simulink subsystem "FuelCellCore"  (R2023b)
settings: Solver=VariableStepAuto  StartTime=0.0  StopTime=10.0  RelTol=1e-3
undefined symbols (not defined in the file): anode_tube_D, cathode_tube_D, comp_rpm_TLU, coolant_num_layers, coolant_num_passes, coolant_tube_D, coolant_w_channels, env_p, env_T, N2_T, radiator_air_area_fins, radiator_air_area_primary, radiator_eta_fin, radiator_N_tubes, radiator_rho, radiator_t_wall, radiator_tube_H, radiator_W, stack_area, stack_iL, stack_mea_rho, stack_num_cells, stack_num_channels, stack_t_gdl, stack_t_membrane, stack_w_channels
libraries: fl_lib x98, nesl_utility_internal x20, slpidlib x2
(part 1 of 3)
settings Model: ModifiedByFormat=The MathWorks, Inc.  Creator=The MathWorks, Inc.  LastModifiedBy=The MathWorks, Inc.
settings SolverCC: MaxZcPerStep=1
settings OptimizationCC: ReuseModelBlockBuffer=off
settings DebuggingCC: UnconnectedInputMsg=warning  UnconnectedOutputMsg=warning  UnconnectedLineMsg=warning  SubsystemReferenceDiagnosticForUnitTest=warning
settings ModelReferenceCC: EnableRefExpFcnMdlSchedulingChecks=on
settings RTWCC: DLArmComputeVersion=19.05

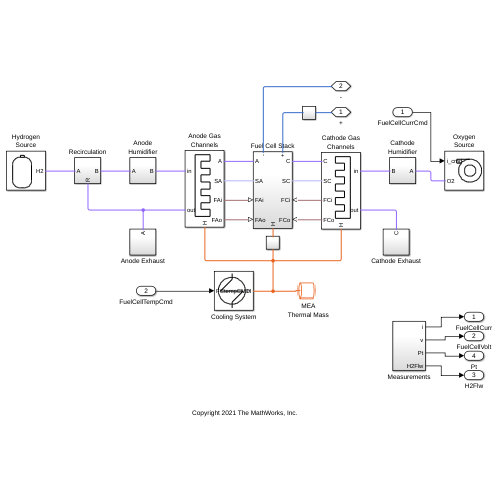
[thumbnail: Simulink's stored preview of the top-level diagram]
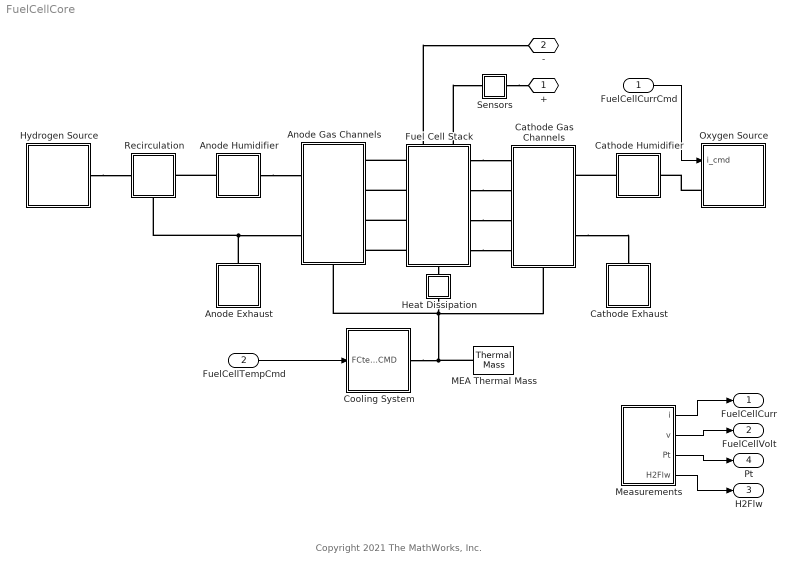
== system FuelCellCore ==
  note: Copyright 2021 The MathWorks, Inc.
  FuelCellCurrCmd : Inport
  FuelCellTempCmd : Inport  Port=2
  Anode Humidifier : Subsystem  Tag=PublishSubsystem
  Anode Exhaust : Subsystem  Tag=PublishSubsystem
      settings: PortSchema="{\"entries\":[{\"content\":{\"sides\":[{\"content\":{\"connectorIds\":[]},\"type\":\"ConnectorPlacement.EquallySpacedRectSide\",\"uuid\":\"6344d1cf-22ea-4a51-9588-07afca0fac15\"},{\"content\":{\"connectorIds\":[],\"side\":\"RIGHT\"},\"type\":\"ConnectorPlacement.EquallySpacedRectSide\",\"uuid\":\"a3908f81-9410-4056-87cd-9faba76d3fb8\"},{\"content\":{\"connectorIds\":[\"LConn1\"],\"side\":\"TOP\"},\"type\":\"ConnectorPlacement.EquallySpacedRectSide\",\"uuid\":\"a1c9e24d-adb9-4361-8e9b-feafccbbdb81\"}]},\"type\":\"ConnectorPlacement.EquallySpacedConnector\",\"uuid\":\"d5180d8f-18a0-491d-9fff-909db43c9aea\"}],\"packageUris\":[\"http://schema.mathworks.com/mf0/Connector/R2020b\"],\"version\":\"1.0\"}"
  Anode Gas Channels : Subsystem  Tag=PublishSubsystem
      settings: PortSchema="{\"entries\":[{\"content\":{\"sides\":[{\"content\":{\"connectorIds\":[\"LConn1\",\"LConn2\"]},\"type\":\"ConnectorPlacement.EquallySpacedRectSide\",\"uuid\":\"f0c92738-2de1-40ac-9e4a-670524600aa2\"},{\"content\":{\"connectorIds\":[\"RConn1\",\"RConn2\",\"RConn3\",\"RConn4\"],\"side\":\"RIGHT\"},\"type\":\"ConnectorPlacement.EquallySpacedRectSide\",\"uuid\":\"f0ed995d-2dce-4bd6-9faa-b1cb502a30b1\"},{\"content\":{\"connectorIds\":[],\"side\":\"TOP\"},\"type\":\"ConnectorPlacement.EquallySpacedRectSide\",\"uuid\":\"b5d2d698-46b6-42b5-a767-bb9f1790aa28\"},{\"content\":{\"connectorIds\":[\"RConn5\"],\"side\":\"BOTTOM\"},\"type\":\"ConnectorPlacement.EquallySpacedRectSide\",\"uuid\":\"3e8c99a3-0044-43a9-bacb-b652445e4ac6\"}]},\"type\":\"ConnectorPlacement.EquallySpacedConnector\",\"uuid\":\"912925fb-ca80-4fe6-8a1d-a2308cfd6f88\"}],\"packageUris\":[\"http://schema.mathworks.com/mf0/Connector/R2020b\"],\"version\":\"1.0\"}"
      mask Display:
      | plot(0, 0)
      | plot(100, 100)
      | 
      | x1 = 25;
      | x2 = 65;
      | y1 = 23;
      | y2 = 95;
      | xt = 15;
      | yt = 9;
      | 
      | x_pattern = [x2 x2    x1+xt x1+xt   x1+xt   x2     ];
      | y_pattern = [y2 y2-yt y2-yt y2-2*yt y2-2*yt y2-2*yt];
      | 
      | plot([x1 x1 x2 x_pattern x_pattern      x_pattern      x_pattern         x2    x1], ...
      |      [y1-yt y2 y2 y_pattern y_pattern-2*yt y_pattern-4*yt y_pattern-6*yt y1-yt y1-yt])
  Cathode Humidifier : Subsystem  Tag=PublishSubsystem
  Cathode Exhaust : Subsystem  Tag=PublishSubsystem
      settings: PortSchema="{\"entries\":[{\"content\":{\"sides\":[{\"content\":{\"connectorIds\":[]},\"type\":\"ConnectorPlacement.EquallySpacedRectSide\",\"uuid\":\"6344d1cf-22ea-4a51-9588-07afca0fac15\"},{\"content\":{\"connectorIds\":[],\"side\":\"RIGHT\"},\"type\":\"ConnectorPlacement.EquallySpacedRectSide\",\"uuid\":\"a3908f81-9410-4056-87cd-9faba76d3fb8\"},{\"content\":{\"connectorIds\":[\"LConn1\"],\"side\":\"TOP\"},\"type\":\"ConnectorPlacement.EquallySpacedRectSide\",\"uuid\":\"a1c9e24d-adb9-4361-8e9b-feafccbbdb81\"}]},\"type\":\"ConnectorPlacement.EquallySpacedConnector\",\"uuid\":\"d5180d8f-18a0-491d-9fff-909db43c9aea\"}],\"packageUris\":[\"http://schema.mathworks.com/mf0/Connector/R2020b\"],\"version\":\"1.0\"}"
  Cathode Gas Channels : Subsystem  Tag=PublishSubsystem
      settings: PortSchema="{\"entries\":[{\"content\":{\"sides\":[{\"content\":{\"connectorIds\":[\"LConn1\",\"LConn2\",\"LConn3\",\"LConn4\"]},\"type\":\"ConnectorPlacement.EquallySpacedRectSide\",\"uuid\":\"d09155df-6760-40de-80f3-d532399b6b43\"},{\"content\":{\"connectorIds\":[\"RConn1\",\"RConn2\"],\"side\":\"RIGHT\"},\"type\":\"ConnectorPlacement.EquallySpacedRectSide\",\"uuid\":\"8f76bd4e-30c2-4c8b-860a-78c10353bd22\"},{\"content\":{\"connectorIds\":[],\"side\":\"TOP\"},\"type\":\"ConnectorPlacement.EquallySpacedRectSide\",\"uuid\":\"7de91a32-4f26-479e-bbec-b6009a288b8f\"},{\"content\":{\"connectorIds\":[\"RConn3\"],\"side\":\"BOTTOM\"},\"type\":\"ConnectorPlacement.EquallySpacedRectSide\",\"uuid\":\"b696b46e-4734-4c8a-bae1-7c8793078c6b\"}]},\"type\":\"ConnectorPlacement.EquallySpacedConnector\",\"uuid\":\"30d7c265-b676-4649-8112-8a94c6c095da\"}],\"packageUris\":[\"http://schema.mathworks.com/mf0/Connector/R2020b\"],\"version\":\"1.0\"}"
      mask Display:
      | plot(0, 0)
      | plot(100, 100)
      | 
      | x1 = 35;
      | x2 = 75;
      | y1 = 23;
      | y2 = 95;
      | xt = 15;
      | yt = 9;
      | 
      | x_pattern = [x1 x1    x2-xt x2-xt   x2-xt   x1     ];
      | y_pattern = [y2 y2-yt y2-yt y2-2*yt y2-2*yt y2-2*yt];
      | 
      | plot([x2 x2 x1 x_pattern x_pattern      x_pattern      x_pattern         x1    x2], ...
      |      [y1-yt y2 y2 y_pattern y_pattern-2*yt y_pattern-4*yt y_pattern-6*yt y1-yt y1-yt])
  Cooling System : Subsystem  Tag=PublishSubsystem
      mask Display:
      | plot(0, 0)
      | plot(100, 100)
      | 
      | n = 80;
      | r = 35;
      | 
      | x = 45;
      | y = 50;
      | t = 5;
      | 
      | plot(cos(linspace(0, 2*pi, n))*r + x, sin(linspace(0, 2*pi, n))*r + y)
      | 
      | plot([x x x-r+t x+r-t x x], [y+r+2*t y+r-t y y y-r+t y-r-2*t])
  Fuel Cell Stack : Subsystem  VariantControl=SSC
      settings: PortSchema="{\"entries\":[{\"content\":{\"sides\":[{\"content\":{\"connectorIds\":[\"LConn1\",\"LConn2\",\"LConn3\",\"LConn4\"]},\"type\":\"ConnectorPlacement.EquallySpacedRectSide\",\"uuid\":\"bdc2282f-c7e2-4f49-b802-006cad4e04a2\"},{\"content\":{\"connectorIds\":[\"RConn1\",\"RConn2\",\"RConn3\",\"RConn4\"],\"side\":\"RIGHT\"},\"type\":\"ConnectorPlacement.EquallySpacedRectSide\",\"uuid\":\"0ce2f163-5da5-49d3-85cb-7045196940f7\"},{\"content\":{\"connectorIds\":[\"LConn5\",\"LConn6\"],\"side\":\"TOP\"},\"type\":\"ConnectorPlacement.EquallySpacedRectSide\",\"uuid\":\"75e1e23b-6ccf-4635-be82-dcdf3f4e1687\"},{\"content\":{\"connectorIds\":[\"RConn5\"],\"side\":\"BOTTOM\"},\"type\":\"ConnectorPlacement.EquallySpacedRectSide\",\"uuid\":\"ec1bdd47-8e50-455a-80ca-a511c9934544\"}]},\"type\":\"ConnectorPlacement.EquallySpacedConnector\",\"uuid\":\"b6082ae9-0c92-40bc-8c32-481d6defd292\"}],\"packageUris\":[\"http://schema.mathworks.com/mf0/Connector/R2020b\"],\"version\":\"1.0\"}"
  Heat Dissipation : Subsystem
      settings: PortSchema="{\"entries\":[{\"content\":{\"sides\":[{\"content\":{\"connectorIds\":[]},\"type\":\"ConnectorPlacement.EquallySpacedRectSide\",\"uuid\":\"40b2385a-b20e-464f-8016-3228e4acac4a\"},{\"content\":{\"connectorIds\":[],\"side\":\"RIGHT\"},\"type\":\"ConnectorPlacement.EquallySpacedRectSide\",\"uuid\":\"0e95dc4b-d2da-4ab6-a6e9-e2cb275776ce\"},{\"content\":{\"connectorIds\":[\"LConn1\"],\"side\":\"TOP\"},\"type\":\"ConnectorPlacement.EquallySpacedRectSide\",\"uuid\":\"0f5995c7-26f6-433d-889b-dea78bcd2b2a\"},{\"content\":{\"connectorIds\":[\"RConn1\"],\"side\":\"BOTTOM\"},\"type\":\"ConnectorPlacement.EquallySpacedRectSide\",\"uuid\":\"a2ee1c19-f9e9-4dbd-a9ff-92feea387e85\"}]},\"type\":\"ConnectorPlacement.EquallySpacedConnector\",\"uuid\":\"721753ea-9ada-4c74-8c6f-50b905d96904\"}],\"packageUris\":[\"http://schema.mathworks.com/mf0/Connector/R2020b\"],\"version\":\"1.0\"}"
  Hydrogen Source : Subsystem  Tag=PublishSubsystem
      mask Display:
      | plot(0, 0)
      | plot(100, 100)
      | 
      | n = 20;
      | r = 20;
      | x1 = 15;
      | x2 = 65;
      | y1 = 5;
      | y2 = 85;
      | 
      | plot([x1 x1], [y1+r y2-r])
      | plot([x1+r x2-r], [y2 y2])
      | plot([x2 x2], [y2-r y1+r])
      | plot([x2-r x1+r], [y1 y1])
      | 
      | plot(cos(linspace(pi/2, pi, n))*r + x1+r, sin(linspace(pi/2, pi, n))*r + y2-r)
      | plot(cos(linspace(0, pi/2, n))*r + x2-r, sin(linspace(0, pi/2, n))*r + y2-r)
      | plot(cos(linspace(3*pi/2, 2*pi, n))*r + x2-r, sin(linspace(3*pi/2, 2*pi, n))*r + y1+r)
      | plot(cos(linspace(pi, 3*pi/2, n))*r + x1+r, sin(linspace(pi, 3*pi/2, n))*r + y1+r)
      | 
      | plot([-5 -5 5 5] + (x1+x2)/2, [0 5 5 0] + y2)
  MEA Thermal Mass : fl_lib/Thermal/Thermal Elements/Thermal Mass  mass_type=foundation.enum.constant_variable.constant  mass=stack_mea_rho * stack_area*1e-4 * (stack_t_membrane + 2*stack_t_gdl)*1e-6 * stack_num_cells kg  sp_heat=stack_mea_cp J/kg/K  mass_min=1e-6 kg  num_ports=foundation.enum.numPorts2.one  m_specify=off  m_priority=High  m=1 kg  m_nominal_specify=off  m_nominal_unit=kg  m_nominal_value=1  T_specify=on  T_priority=High  T=env_T degC  T_nominal_specify=off  T_nominal_unit=K  T_nominal_value=1  Q_specify=off  Q_priority=None  Q=0 W  Q_nominal_specify=off  Q_nominal_unit=W  Q_nominal_value=1
  Measurements : Subsystem
  Oxygen Source : Subsystem  Tag=PublishSubsystem
      mask Display:
      | plot(0, 0)
      | plot(100, 100)
      | 
      | n = 80;
      | r1 = 15;
      | r2 = 30;
      | 
      | plot(cos(linspace(0, 2*pi, n))*r1 + 65, sin(linspace(0, 2*pi, n))*r1 + 50)
      | plot(cos(linspace(0, 2*pi, n))*r2 + 65, sin(linspace(0, 2*pi, n))*r2 + 50)
      | 
      | plot([65 30 30 42], [80 80 70 70])
  Recirculation : Subsystem  Tag=PublishSubsystem
      settings: PortSchema="{\"entries\":[{\"content\":{\"sides\":[{\"content\":{\"connectorIds\":[\"LConn1\"]},\"type\":\"ConnectorPlacement.EquallySpacedRectSide\",\"uuid\":\"a905d28b-4136-4e4b-b56f-ff4ef454860e\"},{\"content\":{\"connectorIds\":[\"RConn1\"],\"side\":\"RIGHT\"},\"type\":\"ConnectorPlacement.EquallySpacedRectSide\",\"uuid\":\"7d453241-460d-4f71-8108-f868ae96b726\"},{\"content\":{\"connectorIds\":[],\"side\":\"TOP\"},\"type\":\"ConnectorPlacement.EquallySpacedRectSide\",\"uuid\":\"5de5a8e7-eaa9-43ea-9e3e-e109b24be5c4\"},{\"content\":{\"connectorIds\":[\"RConn2\"],\"side\":\"BOTTOM\"},\"type\":\"ConnectorPlacement.EquallySpacedRectSide\",\"uuid\":\"9c44ad98-d3d2-40d8-a226-ad16e20687d9\"}]},\"type\":\"ConnectorPlacement.EquallySpacedConnector\",\"uuid\":\"be431bc9-ad83-41b5-a4a3-7fe11e97fedb\"}],\"packageUris\":[\"http://schema.mathworks.com/mf0/Connector/R2020b\"],\"version\":\"1.0\"}"
  Sensors : Subsystem
      settings: PortSchema="{\"entries\":[{\"content\":{\"sides\":[{\"content\":{\"connectorIds\":[]},\"type\":\"ConnectorPlacement.EquallySpacedRectSide\",\"uuid\":\"40b2385a-b20e-464f-8016-3228e4acac4a\"},{\"content\":{\"connectorIds\":[],\"side\":\"RIGHT\"},\"type\":\"ConnectorPlacement.EquallySpacedRectSide\",\"uuid\":\"0e95dc4b-d2da-4ab6-a6e9-e2cb275776ce\"},{\"content\":{\"connectorIds\":[\"LConn1\"],\"side\":\"TOP\"},\"type\":\"ConnectorPlacement.EquallySpacedRectSide\",\"uuid\":\"0f5995c7-26f6-433d-889b-dea78bcd2b2a\"},{\"content\":{\"connectorIds\":[\"RConn1\"],\"side\":\"BOTTOM\"},\"type\":\"ConnectorPlacement.EquallySpacedRectSide\",\"uuid\":\"a2ee1c19-f9e9-4dbd-a9ff-92feea387e85\"}]},\"type\":\"ConnectorPlacement.EquallySpacedConnector\",\"uuid\":\"721753ea-9ada-4c74-8c6f-50b905d96904\"}],\"packageUris\":[\"http://schema.mathworks.com/mf0/Connector/R2020b\"],\"version\":\"1.0\"}"
  + : PMIOPort  Side=Right
  - : PMIOPort  Port=2  Side=Right
  FuelCellCurr : Outport
  FuelCellVolt : Outport  Port=2
  H2Flw : Outport  Port=3
  Pt : Outport  Port=4
  wires:
  Measurements/1(i) -> FuelCellCurr/1
  FuelCellCurrCmd/1 -> Oxygen Source/1(i_cmd)
  FuelCellTempCmd/1 -> Cooling System/1(FCtempCMD)
  Measurements/2(v) -> FuelCellVolt/1
  Measurements/3(Pt) -> Pt/1
  Measurements/4(H2Flw) -> H2Flw/1
  connections:
  Anode Exhaust/LConn1 -- Recirculation/RConn2 -- Anode Gas Channels/LConn2
  Heat Dissipation/RConn1 -- MEA Thermal Mass/LConn1 -- Cooling System/RConn1 -- Anode Gas Channels/RConn5 -- Cathode Gas Channels/RConn3
  Fuel Cell Stack/LConn2 -- Anode Gas Channels/RConn2
  Hydrogen Source/RConn1 -- Recirculation/LConn1
  Fuel Cell Stack/LConn3 -- Anode Gas Channels/RConn3
  Fuel Cell Stack/RConn1 -- Cathode Gas Channels/LConn1
  Cathode Humidifier/LConn1 -- Cathode Gas Channels/RConn1
  Sensors/RConn1 -- +/RConn1
  Fuel Cell Stack/RConn2 -- Cathode Gas Channels/LConn2
  Cathode Gas Channels/RConn2 -- Cathode Exhaust/LConn1
  Fuel Cell Stack/RConn4 -- Cathode Gas Channels/LConn4
  Fuel Cell Stack/RConn3 -- Cathode Gas Channels/LConn3
  Oxygen Source/LConn1 -- Cathode Humidifier/RConn1
  Anode Humidifier/LConn1 -- Recirculation/RConn1
  Fuel Cell Stack/LConn5 -- -/RConn1
  Fuel Cell Stack/RConn5 -- Heat Dissipation/LConn1
  Fuel Cell Stack/LConn1 -- Anode Gas Channels/RConn1
  Anode Humidifier/RConn1 -- Anode Gas Channels/LConn1
  Fuel Cell Stack/LConn4 -- Anode Gas Channels/RConn4
  Fuel Cell Stack/LConn6 -- Sensors/LConn1

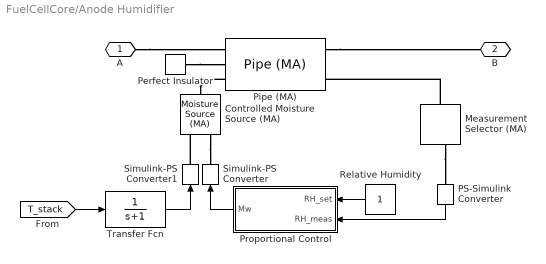
== system FuelCellCore/Anode Humidifier ==
  Controlled Moisture Source (MA) : fl_lib/Moist Air/Sources/Moisture & Trace Gas Sources/Moisture Source (MA)  source_type=foundation.enum.constant_controlled.controlled  moisture_source_spec=foundation.enum.moisture_source_spec.vapor  moisture_mass_flow=0 kg/s  temperature_spec=foundation.enum.temperature_spec.atmospheric  moisture_temperature=293.15 K  Phi_S_specify=off  Phi_S_priority=None  Phi_S=0 kW  Phi_S_nominal_specify=off  Phi_S_nominal_unit=kW  Phi_S_nominal_value=1  mdot_w_S_specify=off  mdot_w_S_priority=None  mdot_w_S=0 kg/s  mdot_w_S_nominal_specify=off  mdot_w_S_nominal_unit=kg/s  mdot_w_S_nominal_value=1
      settings: InternalSimscapePortConfiguration="{\"Bottom\":[],\"Left\":[{\"id\":\"S\",\"label\":\"S\",\"type\":\"foundation.moist_air.moist_air_source\"}],\"Right\":[{\"id\":\"M\",\"label\":\"M\",\"type\":\"input\"},{\"id\":\"T\",\"label\":\"T\",\"type\":\"input\"}],\"Top\":[]}"
  Measurement Selector (MA) : fl_lib/Moist Air/Sensors/Measurement Selector (MA)  moisture_spec=foundation.enum.moisture_spec.relative_humidity  trace_gas_spec=foundation.enum.trace_gas_spec.mole_fraction
  PS-Simulink Converter : nesl_utility_internal/PS-Simulink Converter  PhysicalDomain=network_engine_domain  SubClassName=ps_output  LeftPortType=input  RightPortType=output  PseudoPeriodic=off  Frequencies=[]  VectorFormat=1-D array  Unit=1  AffineConversion=off
  Perfect Insulator : fl_lib/Thermal/Thermal Elements/Perfect Insulator  T_specify=off  T_priority=None  T=0 K  T_nominal_specify=off  T_nominal_unit=K  T_nominal_value=1
  Pipe (MA) : fl_lib/Moist Air/Elements/Pipe (MA)  length=0.25 m  area=pi*0.05^2/4 m^2  Dh=0.05 m  length_add=0.1 m  roughness=15e-6 m  Re_lam=2000  Re_tur=4000  shape_factor=64  Nu_lam=3.66  wall_condensation=simscape.enum.onoff.off  RH_ws=1  time_constant=1e-3 s  moisture_trace_gas_source=foundation.enum.moisture_trace_gas_source.controlled  moisture_source_spec=foundation.enum.moisture_source_spec.vapor  moisture_mass_flow=0 kg/s  moisture_temperature_spec=foundation.enum.temperature_spec.atmospheric  moisture_temperature=293.15 K  trace_gas_mass_flow=0 kg/s  trace_gas_temperature_spec=foundation.enum.temperature_spec.atmospheric  trace_gas_temperature=293.15 K  p_I_specify=on  p_I_priority=High  p_I=env_p MPa  p_I_nominal_specify=off  p_I_nominal_unit=MPa  p_I_nominal_value=1  T_I_specify=on  T_I_priority=High  T_I=env_T degC  T_I_nominal_specify=off  T_I_nominal_unit=K  T_I_nominal_value=1  RH_I_specify=off  RH_I_priority=High  RH_I=0  RH_I_nominal_specify=off  RH_I_nominal_unit=1  RH_I_nominal_value=1  x_w_I_specify=off  x_w_I_priority=None  x_w_I=0  x_w_I_nominal_specify=off  x_w_I_nominal_unit=1  x_w_I_nominal_value=1  y_w_I_specify=off  y_w_I_priority=None  y_w_I=0  y_w_I_nominal_specify=off  y_w_I_nominal_unit=1  y_w_I_nominal_value=1  HR_I_specify=off  HR_I_priority=None  HR_I=0  HR_I_nominal_specify=off  HR_I_nominal_unit=1  HR_I_nominal_value=1  x_g_I_specify=on  x_g_I_priority=None  x_g_I=0  x_g_I_nominal_specify=off  x_g_I_nominal_unit=1  x_g_I_nominal_value=1  y_g_I_specify=on  y_g_I_priority=High  y_g_I=tank_yH2  y_g_I_nominal_specify=off  y_g_I_nominal_unit=1  y_g_I_nominal_value=1
      settings: InternalSimscapePortConfiguration="{\"Bottom\":[],\"Left\":[{\"id\":\"A\",\"label\":\"A\",\"type\":\"foundation.moist_air.moist_air\"},{\"id\":\"H\",\"label\":\"H\",\"type\":\"foundation.thermal.thermal\"},{\"id\":\"S\",\"label\":\"S\",\"type\":\"foundation.moist_air.moist_air_source\"}],\"Right\":[{\"id\":\"B\",\"label\":\"B\",\"type\":\"foundation.moist_air.moist_air\"},{\"id\":\"W\",\"label\":\"W\",\"type\":\"output\"},{\"id\":\"F\",\"label\":\"F\",\"type\":\"output\"}],\"Top\":[]}"
  Proportional Control : Subsystem
  Relative Humidity : Constant  SampleTime=-1
  Simulink-PS Converter : nesl_utility_internal/Simulink-PS Converter  PhysicalDomain=network_engine_domain  SubClassName=ps_input  LeftPortType=input  RightPortType=output  PseudoPeriodic=off  Frequencies=[]  NoiseDistribution=none  NoiseParameters=[]  Unit=kg/s  AffineConversion=off  FilteringAndDerivatives=provide  SimscapeFilterOrder=1  InputFilterTimeConstant=0.001  UdotUserProvided=0
  Simulink-PS Converter1 : nesl_utility_internal/Simulink-PS Converter  PhysicalDomain=network_engine_domain  SubClassName=ps_input  LeftPortType=input  RightPortType=output  PseudoPeriodic=off  Frequencies=[]  NoiseDistribution=none  NoiseParameters=[]  Unit=degC  AffineConversion=on  FilteringAndDerivatives=provide  SimscapeFilterOrder=1  InputFilterTimeConstant=0.001  UdotUserProvided=0
  Transfer Fcn : TransferFcn  Denominator=[1 1]
  A : PMIOPort  Side=Left
  B : PMIOPort  Port=2  Side=Right
  wires:
  Transfer Fcn/1 -> Simulink-PS Converter1/1
  [T_stack] -> Transfer Fcn/1
  Relative Humidity/1 -> Proportional Control/1(RH_set)
  PS-Simulink Converter/1 -> Proportional Control/2(RH_meas)
  Proportional Control/1(Mw) -> Simulink-PS Converter/1
  connections:
  Controlled Moisture Source (MA)/RConn1 -- Simulink-PS Converter/RConn1
  Measurement Selector (MA)/LConn1 -- Pipe (MA)/RConn3
  Simulink-PS Converter1/RConn1 -- Controlled Moisture Source (MA)/RConn2
  Pipe (MA)/LConn3 -- Controlled Moisture Source (MA)/LConn1
  Perfect Insulator/LConn1 -- Pipe (MA)/LConn2
  Pipe (MA)/RConn1 -- B/RConn1
  A/RConn1 -- Pipe (MA)/LConn1
  Measurement Selector (MA)/RConn3 -- PS-Simulink Converter/LConn1

== system FuelCellCore/Anode Exhaust ==
  Constant : Constant  Value=0  SampleTime=-1
  Convective Heat Transfer : fl_lib/Thermal/Thermal Elements/Convective Heat Transfer  thermal_type=foundation.enum.constant_variable.constant  area=pi*anode_tube_D*1 m^2  heat_tr_coeff=20 W/(m^2 * K)  min_heat_tr_coeff=1e-3 W/(K*m^2)  T_specify=off  T_priority=None  T=0 K  T_nominal_specify=off  T_nominal_unit=K  T_nominal_value=1  Q_specify=off  Q_priority=None  Q=0 W  Q_nominal_specify=off  Q_nominal_unit=W  Q_nominal_value=1
  Environment : fl_lib/Moist Air/Elements/Reservoir (MA)  pressure_spec=foundation.enum.pressure_spec.specified  reservoir_pressure=env_p MPa  temperature_spec=foundation.enum.temperature_spec.specified  reservoir_temperature=env_T degC  moisture_spec=foundation.enum.moisture_spec.relative_humidity  reservoir_RH=0  reservoir_x_w=0.01  reservoir_y_w=0.01  reservoir_HR=0.01  reservoir_Tw=287 K  trace_gas_spec=foundation.enum.trace_gas_spec.mole_fraction  reservoir_x_g=0.001  reservoir_y_g=tank_yH2  RH_ws=1  area_A=pi*anode_tube_D^2/4 m^2
  Environment Temperature : fl_lib/Thermal/Thermal Sources/Temperature Source  temperature=env_T degC
  Max Area : fl_lib/Physical Signals/Functions/PS Gain  gain=pi*(0.2*anode_tube_D)^2/4 m^2
  Pipe (MA) : fl_lib/Moist Air/Elements/Pipe (MA)  length=1 m  area=pi*anode_tube_D^2/4 m^2  Dh=anode_tube_D m  length_add=0.1 m  roughness=15e-6 m  Re_lam=2000  Re_tur=4000  shape_factor=64  Nu_lam=3.66  wall_condensation=simscape.enum.onoff.off  RH_ws=1  time_constant=1e-3 s  moisture_trace_gas_source=foundation.enum.moisture_trace_gas_source.none  moisture_source_spec=foundation.enum.moisture_source_spec.vapor  moisture_mass_flow=0 kg/s  moisture_temperature_spec=foundation.enum.temperature_spec.atmospheric  moisture_temperature=293.15 K  trace_gas_mass_flow=0 kg/s  trace_gas_temperature_spec=foundation.enum.temperature_spec.atmospheric  trace_gas_temperature=293.15 K  p_I_specify=on  p_I_priority=High  p_I=env_p MPa  p_I_nominal_specify=off  p_I_nominal_unit=MPa  p_I_nominal_value=1  T_I_specify=on  T_I_priority=High  T_I=env_T degC  T_I_nominal_specify=off  T_I_nominal_unit=K  T_I_nominal_value=1  RH_I_specify=off  RH_I_priority=High  RH_I=0  RH_I_nominal_specify=off  RH_I_nominal_unit=1  RH_I_nominal_value=1  x_w_I_specify=off  x_w_I_priority=None  x_w_I=0  x_w_I_nominal_specify=off  x_w_I_nominal_unit=1  x_w_I_nominal_value=1  y_w_I_specify=off  y_w_I_priority=None  y_w_I=0  y_w_I_nominal_specify=off  y_w_I_nominal_unit=1  y_w_I_nominal_value=1  HR_I_specify=off  HR_I_priority=None  HR_I=0  HR_I_nominal_specify=off  HR_I_nominal_unit=1  HR_I_nominal_value=1  x_g_I_specify=on  x_g_I_priority=None  x_g_I=0  x_g_I_nominal_specify=off  x_g_I_nominal_unit=1  x_g_I_nominal_value=1  y_g_I_specify=on  y_g_I_priority=High  y_g_I=tank_yH2  y_g_I_nominal_specify=off  y_g_I_nominal_unit=1  y_g_I_nominal_value=1
  Purge Valve : fl_lib/Moist Air/Elements/Local Restriction (MA)  restriction_type=foundation.enum.restriction_type.variable  restriction_area=0.001 m^2  min_area=pi*(1e-4*anode_tube_D)^2/4 m^2  max_area=pi*(0.2*anode_tube_D)^2/4 m^2  area=pi*anode_tube_D^2/4 m^2  Cd=0.64  B_lam=0.999
  Simulink-PS Converter : nesl_utility_internal/Simulink-PS Converter  PhysicalDomain=network_engine_domain  SubClassName=ps_input  LeftPortType=input  RightPortType=output  PseudoPeriodic=off  Frequencies=[]  NoiseDistribution=none  NoiseParameters=[]  Unit=1  AffineConversion=off  FilteringAndDerivatives=provide  SimscapeFilterOrder=1  InputFilterTimeConstant=0.001  UdotUserProvided=0
  Transfer Fcn : TransferFcn  Denominator=[1 1]
  A : PMIOPort  Side=Left
  wires:
  Constant/1 -> Transfer Fcn/1
  Transfer Fcn/1 -> Simulink-PS Converter/1
  connections:
  Environment/LConn1 -- Purge Valve/RConn1
  A/RConn1 -- Pipe (MA)/LConn1
  Purge Valve/LConn1 -- Pipe (MA)/RConn1
  Simulink-PS Converter/RConn1 -- Max Area/LConn1
  Max Area/RConn1 -- Purge Valve/LConn2
  Convective Heat Transfer/LConn1 -- Pipe (MA)/LConn2
  Environment Temperature/LConn1 -- Convective Heat Transfer/RConn1

== system FuelCellCore/Anode Gas Channels ==
  Pipe (MA) : fl_lib/Moist Air/Elements/Pipe (MA)  length=sqrt(stack_area) / 2 cm  area=stack_w_channels^2 * stack_num_channels * stack_num_cells cm^2  Dh=stack_w_channels cm  length_add=1 cm  roughness=15e-6 m  Re_lam=2000  Re_tur=4000  shape_factor=64  Nu_lam=3.66  wall_condensation=simscape.enum.onoff.off  RH_ws=1  time_constant=1e-3 s  moisture_trace_gas_source=foundation.enum.moisture_trace_gas_source.none  moisture_source_spec=foundation.enum.moisture_source_spec.vapor  moisture_mass_flow=0 kg/s  moisture_temperature_spec=foundation.enum.temperature_spec.atmospheric  moisture_temperature=293.15 K  trace_gas_mass_flow=0 kg/s  trace_gas_temperature_spec=foundation.enum.temperature_spec.atmospheric  trace_gas_temperature=293.15 K  p_I_specify=on  p_I_priority=High  p_I=env_p MPa  p_I_nominal_specify=off  p_I_nominal_unit=MPa  p_I_nominal_value=1  T_I_specify=on  T_I_priority=High  T_I=env_T degC  T_I_nominal_specify=off  T_I_nominal_unit=K  T_I_nominal_value=1  RH_I_specify=off  RH_I_priority=High  RH_I=0  RH_I_nominal_specify=off  RH_I_nominal_unit=1  RH_I_nominal_value=1  x_w_I_specify=off  x_w_I_priority=None  x_w_I=0  x_w_I_nominal_specify=off  x_w_I_nominal_unit=1  x_w_I_nominal_value=1  y_w_I_specify=off  y_w_I_priority=None  y_w_I=0  y_w_I_nominal_specify=off  y_w_I_nominal_unit=1  y_w_I_nominal_value=1  HR_I_specify=off  HR_I_priority=None  HR_I=0  HR_I_nominal_specify=off  HR_I_nominal_unit=1  HR_I_nominal_value=1  x_g_I_specify=on  x_g_I_priority=None  x_g_I=0  x_g_I_nominal_specify=off  x_g_I_nominal_unit=1  x_g_I_nominal_value=1  y_g_I_specify=on  y_g_I_priority=High  y_g_I=tank_yH2  y_g_I_nominal_specify=off  y_g_I_nominal_unit=1  y_g_I_nominal_value=1
  Pipe (MA)1 : fl_lib/Moist Air/Elements/Pipe (MA)  length=sqrt(stack_area) / 2 cm  area=stack_w_channels^2 * stack_num_channels * stack_num_cells cm^2  Dh=stack_w_channels cm  length_add=1 cm  roughness=15e-6 m  Re_lam=2000  Re_tur=4000  shape_factor=64  Nu_lam=3.66  wall_condensation=simscape.enum.onoff.off  RH_ws=1  time_constant=1e-3 s  moisture_trace_gas_source=foundation.enum.moisture_trace_gas_source.controlled  moisture_source_spec=foundation.enum.moisture_source_spec.vapor  moisture_mass_flow=0 kg/s  moisture_temperature_spec=foundation.enum.temperature_spec.atmospheric  moisture_temperature=293.15 K  trace_gas_mass_flow=0 kg/s  trace_gas_temperature_spec=foundation.enum.temperature_spec.atmospheric  trace_gas_temperature=293.15 K  p_I_specify=on  p_I_priority=High  p_I=env_p MPa  p_I_nominal_specify=off  p_I_nominal_unit=MPa  p_I_nominal_value=1  T_I_specify=on  T_I_priority=High  T_I=env_T degC  T_I_nominal_specify=off  T_I_nominal_unit=K  T_I_nominal_value=1  RH_I_specify=off  RH_I_priority=High  RH_I=0  RH_I_nominal_specify=off  RH_I_nominal_unit=1  RH_I_nominal_value=1  x_w_I_specify=off  x_w_I_priority=None  x_w_I=0  x_w_I_nominal_specify=off  x_w_I_nominal_unit=1  x_w_I_nominal_value=1  y_w_I_specify=off  y_w_I_priority=None  y_w_I=0  y_w_I_nominal_specify=off  y_w_I_nominal_unit=1  y_w_I_nominal_value=1  HR_I_specify=off  HR_I_priority=None  HR_I=0  HR_I_nominal_specify=off  HR_I_nominal_unit=1  HR_I_nominal_value=1  x_g_I_specify=on  x_g_I_priority=None  x_g_I=0  x_g_I_nominal_specify=off  x_g_I_nominal_unit=1  x_g_I_nominal_value=1  y_g_I_specify=on  y_g_I_priority=High  y_g_I=tank_yH2  y_g_I_nominal_specify=off  y_g_I_nominal_unit=1  y_g_I_nominal_value=1
      settings: InternalSimscapePortConfiguration="{\"Bottom\":[],\"Left\":[{\"id\":\"A\",\"label\":\"A\",\"type\":\"foundation.moist_air.moist_air\"},{\"id\":\"H\",\"label\":\"H\",\"type\":\"foundation.thermal.thermal\"},{\"id\":\"S\",\"label\":\"S\",\"type\":\"foundation.moist_air.moist_air_source\"}],\"Right\":[{\"id\":\"B\",\"label\":\"B\",\"type\":\"foundation.moist_air.moist_air\"},{\"id\":\"W\",\"label\":\"W\",\"type\":\"output\"},{\"id\":\"F\",\"label\":\"F\",\"type\":\"output\"}],\"Top\":[]}"
  in : PMIOPort  Side=Left
  out : PMIOPort  Port=2  Side=Left
  A : PMIOPort  Port=3  Side=Right
  SA : PMIOPort  Port=4  Side=Right
  FAi : PMIOPort  Port=5  Side=Right
  FAo : PMIOPort  Port=6  Side=Right
  H : PMIOPort  Port=7  Side=Right
  connections:
  Pipe (MA)/LConn1 -- in/RConn1
  Pipe (MA)1/RConn1 -- out/RConn1
  Pipe (MA)/LConn2 -- Pipe (MA)1/LConn2 -- H/RConn1
  FAo/RConn1 -- Pipe (MA)1/RConn3
  Pipe (MA)/RConn3 -- FAi/RConn1
  Pipe (MA)1/LConn3 -- SA/RConn1
  Pipe (MA)/RConn1 -- Pipe (MA)1/LConn1 -- A/RConn1

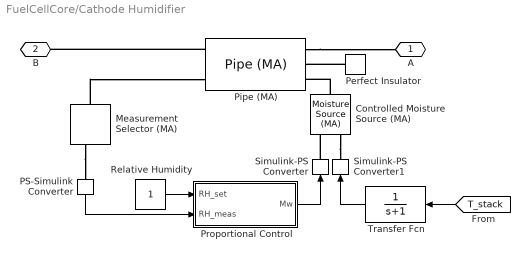
== system FuelCellCore/Cathode Humidifier ==
  Controlled Moisture Source (MA) : fl_lib/Moist Air/Sources/Moisture & Trace Gas Sources/Moisture Source (MA)  source_type=foundation.enum.constant_controlled.controlled  moisture_source_spec=foundation.enum.moisture_source_spec.vapor  moisture_mass_flow=0 kg/s  temperature_spec=foundation.enum.temperature_spec.atmospheric  moisture_temperature=293.15 K  Phi_S_specify=off  Phi_S_priority=None  Phi_S=0 kW  Phi_S_nominal_specify=off  Phi_S_nominal_unit=kW  Phi_S_nominal_value=1  mdot_w_S_specify=off  mdot_w_S_priority=None  mdot_w_S=0 kg/s  mdot_w_S_nominal_specify=off  mdot_w_S_nominal_unit=kg/s  mdot_w_S_nominal_value=1
      settings: InternalSimscapePortConfiguration="{\"Bottom\":[],\"Left\":[{\"id\":\"S\",\"label\":\"S\",\"type\":\"foundation.moist_air.moist_air_source\"}],\"Right\":[{\"id\":\"M\",\"label\":\"M\",\"type\":\"input\"},{\"id\":\"T\",\"label\":\"T\",\"type\":\"input\"}],\"Top\":[]}"
  Measurement Selector (MA) : fl_lib/Moist Air/Sensors/Measurement Selector (MA)  moisture_spec=foundation.enum.moisture_spec.relative_humidity  trace_gas_spec=foundation.enum.trace_gas_spec.mole_fraction
  PS-Simulink Converter : nesl_utility_internal/PS-Simulink Converter  PhysicalDomain=network_engine_domain  SubClassName=ps_output  LeftPortType=input  RightPortType=output  PseudoPeriodic=off  Frequencies=[]  VectorFormat=1-D array  Unit=1  AffineConversion=off
  Perfect Insulator : fl_lib/Thermal/Thermal Elements/Perfect Insulator  T_specify=off  T_priority=None  T=0 K  T_nominal_specify=off  T_nominal_unit=K  T_nominal_value=1
  Pipe (MA) : fl_lib/Moist Air/Elements/Pipe (MA)  length=0.25 m  area=pi*0.05^2/4 m^2  Dh=0.05 m  length_add=0.1 m  roughness=15e-6 m  Re_lam=2000  Re_tur=4000  shape_factor=64  Nu_lam=3.66  wall_condensation=simscape.enum.onoff.off  RH_ws=1  time_constant=1e-3 s  moisture_trace_gas_source=foundation.enum.moisture_trace_gas_source.controlled  moisture_source_spec=foundation.enum.moisture_source_spec.vapor  moisture_mass_flow=0 kg/s  moisture_temperature_spec=foundation.enum.temperature_spec.atmospheric  moisture_temperature=293.15 K  trace_gas_mass_flow=0 kg/s  trace_gas_temperature_spec=foundation.enum.temperature_spec.atmospheric  trace_gas_temperature=293.15 K  p_I_specify=on  p_I_priority=High  p_I=env_p MPa  p_I_nominal_specify=off  p_I_nominal_unit=MPa  p_I_nominal_value=1  T_I_specify=on  T_I_priority=High  T_I=env_T degC  T_I_nominal_specify=off  T_I_nominal_unit=K  T_I_nominal_value=1  RH_I_specify=on  RH_I_priority=High  RH_I=env_RH  RH_I_nominal_specify=off  RH_I_nominal_unit=1  RH_I_nominal_value=1  x_w_I_specify=off  x_w_I_priority=None  x_w_I=0  x_w_I_nominal_specify=off  x_w_I_nominal_unit=1  x_w_I_nominal_value=1  y_w_I_specify=off  y_w_I_priority=None  y_w_I=0  y_w_I_nominal_specify=off  y_w_I_nominal_unit=1  y_w_I_nominal_value=1  HR_I_specify=off  HR_I_priority=None  HR_I=0  HR_I_nominal_specify=off  HR_I_nominal_unit=1  HR_I_nominal_value=1  x_g_I_specify=on  x_g_I_priority=None  x_g_I=0  x_g_I_nominal_specify=off  x_g_I_nominal_unit=1  x_g_I_nominal_value=1  y_g_I_specify=on  y_g_I_priority=High  y_g_I=env_yO2  y_g_I_nominal_specify=off  y_g_I_nominal_unit=1  y_g_I_nominal_value=1
      settings: InternalSimscapePortConfiguration="{\"Bottom\":[],\"Left\":[{\"id\":\"A\",\"label\":\"A\",\"type\":\"foundation.moist_air.moist_air\"},{\"id\":\"H\",\"label\":\"H\",\"type\":\"foundation.thermal.thermal\"},{\"id\":\"S\",\"label\":\"S\",\"type\":\"foundation.moist_air.moist_air_source\"}],\"Right\":[{\"id\":\"B\",\"label\":\"B\",\"type\":\"foundation.moist_air.moist_air\"},{\"id\":\"W\",\"label\":\"W\",\"type\":\"output\"},{\"id\":\"F\",\"label\":\"F\",\"type\":\"output\"}],\"Top\":[]}"
  Proportional Control : Subsystem
  Relative Humidity : Constant  SampleTime=-1
  Simulink-PS Converter : nesl_utility_internal/Simulink-PS Converter  PhysicalDomain=network_engine_domain  SubClassName=ps_input  LeftPortType=input  RightPortType=output  PseudoPeriodic=off  Frequencies=[]  NoiseDistribution=none  NoiseParameters=[]  Unit=kg/s  AffineConversion=off  FilteringAndDerivatives=provide  SimscapeFilterOrder=1  InputFilterTimeConstant=0.001  UdotUserProvided=0
  Simulink-PS Converter1 : nesl_utility_internal/Simulink-PS Converter  PhysicalDomain=network_engine_domain  SubClassName=ps_input  LeftPortType=input  RightPortType=output  PseudoPeriodic=off  Frequencies=[]  NoiseDistribution=none  NoiseParameters=[]  Unit=degC  AffineConversion=on  FilteringAndDerivatives=provide  SimscapeFilterOrder=1  InputFilterTimeConstant=0.001  UdotUserProvided=0
  Transfer Fcn : TransferFcn  Denominator=[1 1]
  A : PMIOPort  Side=Right
  B : PMIOPort  Port=2  Side=Left
  wires:
  Transfer Fcn/1 -> Simulink-PS Converter1/1
  [T_stack] -> Transfer Fcn/1
  Proportional Control/1(Mw) -> Simulink-PS Converter/1
  Relative Humidity/1 -> Proportional Control/1(RH_set)
  PS-Simulink Converter/1 -> Proportional Control/2(RH_meas)
  connections:
  Controlled Moisture Source (MA)/RConn2 -- Simulink-PS Converter1/RConn1
  Measurement Selector (MA)/LConn1 -- Pipe (MA)/RConn3
  Simulink-PS Converter/RConn1 -- Controlled Moisture Source (MA)/RConn1
  Perfect Insulator/LConn1 -- Pipe (MA)/LConn2
  Measurement Selector (MA)/RConn3 -- PS-Simulink Converter/LConn1
  Controlled Moisture Source (MA)/LConn1 -- Pipe (MA)/LConn3
  Pipe (MA)/RConn1 -- B/RConn1
  Pipe (MA)/LConn1 -- A/RConn1

== system FuelCellCore/Cathode Exhaust ==
  Constant1 : Constant  Value=env_p  SampleTime=-1
  Convective Heat Transfer : fl_lib/Thermal/Thermal Elements/Convective Heat Transfer  thermal_type=foundation.enum.constant_variable.constant  area=pi*cathode_tube_D*1 m^2  heat_tr_coeff=20 W/(m^2 * K)  min_heat_tr_coeff=1e-3 W/(K*m^2)  T_specify=off  T_priority=None  T=0 K  T_nominal_specify=off  T_nominal_unit=K  T_nominal_value=1  Q_specify=off  Q_priority=None  Q=0 W  Q_nominal_specify=off  Q_nominal_unit=W  Q_nominal_value=1
  Environment : fl_lib/Moist Air/Elements/Reservoir (MA)  pressure_spec=foundation.enum.pressure_spec.specified  reservoir_pressure=env_p MPa  temperature_spec=foundation.enum.temperature_spec.specified  reservoir_temperature=env_T degC  moisture_spec=foundation.enum.moisture_spec.relative_humidity  reservoir_RH=env_RH  reservoir_x_w=0.01  reservoir_y_w=0.01  reservoir_HR=0.01  reservoir_Tw=287 K  trace_gas_spec=foundation.enum.trace_gas_spec.mole_fraction  reservoir_x_g=0.001  reservoir_y_g=env_yO2  RH_ws=1  area_A=pi*cathode_tube_D^2/4 m^2
  Environment Temperature : fl_lib/Thermal/Thermal Sources/Temperature Source  temperature=env_T degC
  Pipe (MA) : fl_lib/Moist Air/Elements/Pipe (MA)  length=1 m  area=pi*cathode_tube_D^2/4 m^2  Dh=cathode_tube_D m  length_add=0.1 m  roughness=15e-6 m  Re_lam=2000  Re_tur=4000  shape_factor=64  Nu_lam=3.66  wall_condensation=simscape.enum.onoff.off  RH_ws=1  time_constant=1e-3 s  moisture_trace_gas_source=foundation.enum.moisture_trace_gas_source.none  moisture_source_spec=foundation.enum.moisture_source_spec.vapor  moisture_mass_flow=0 kg/s  moisture_temperature_spec=foundation.enum.temperature_spec.atmospheric  moisture_temperature=293.15 K  trace_gas_mass_flow=0 kg/s  trace_gas_temperature_spec=foundation.enum.temperature_spec.atmospheric  trace_gas_temperature=293.15 K  p_I_specify=on  p_I_priority=High  p_I=env_p MPa  p_I_nominal_specify=off  p_I_nominal_unit=MPa  p_I_nominal_value=1  T_I_specify=on  T_I_priority=High  T_I=env_T degC  T_I_nominal_specify=off  T_I_nominal_unit=K  T_I_nominal_value=1  RH_I_specify=on  RH_I_priority=High  RH_I=env_RH  RH_I_nominal_specify=off  RH_I_nominal_unit=1  RH_I_nominal_value=1  x_w_I_specify=off  x_w_I_priority=None  x_w_I=0  x_w_I_nominal_specify=off  x_w_I_nominal_unit=1  x_w_I_nominal_value=1  y_w_I_specify=off  y_w_I_priority=None  y_w_I=0  y_w_I_nominal_specify=off  y_w_I_nominal_unit=1  y_w_I_nominal_value=1  HR_I_specify=off  HR_I_priority=None  HR_I=0  HR_I_nominal_specify=off  HR_I_nominal_unit=1  HR_I_nominal_value=1  x_g_I_specify=on  x_g_I_priority=None  x_g_I=0  x_g_I_nominal_specify=off  x_g_I_nominal_unit=1  x_g_I_nominal_value=1  y_g_I_specify=on  y_g_I_priority=High  y_g_I=env_yO2  y_g_I_nominal_specify=off  y_g_I_nominal_unit=1  y_g_I_nominal_value=1
  Pressure Relief Valve : Subsystem  Tag=PublishSubsystem  mask(Pressure Relief Valve){D=cathode_tube_D, r_min=1e-4, r_max=0.8, p_range=0.005}
      mask prompts: D "Connecting tube diameter (m)"; r_min "Min diameter ratio"; r_max "Max diameter ratio"; p_range "Pressure regulation range (MPa)"
      mask help: This subsystem models a pressure relief valve that maintains a set pressure at port A. The valve is normally closed. When the pressure is above the set pressure, it begins to open.
  Simulink-PS Converter : nesl_utility_internal/Simulink-PS Converter  PhysicalDomain=network_engine_domain  SubClassName=ps_input  LeftPortType=input  RightPortType=output  PseudoPeriodic=off  Frequencies=[]  NoiseDistribution=none  NoiseParameters=[]  Unit=MPa  AffineConversion=off  FilteringAndDerivatives=provide  SimscapeFilterOrder=1  InputFilterTimeConstant=0.001  UdotUserProvided=0
  Stack Pressure : Constant  Value=0.06  SampleTime=-1
  Sum : Sum  Inputs=++|
  C : PMIOPort  Side=Left
  wires:
  Stack Pressure/1 -> Sum/1
  Sum/1 -> Simulink-PS Converter/1
  Constant1/1 -> Sum/2
  connections:
  Pipe (MA)/RConn1 -- Pressure Relief Valve/LConn1
  C/RConn1 -- Pipe (MA)/LConn1
  Convective Heat Transfer/LConn1 -- Pipe (MA)/LConn2
  Environment Temperature/LConn1 -- Convective Heat Transfer/RConn1
  Pressure Relief Valve/RConn1 -- Environment/LConn1
  Simulink-PS Converter/RConn1 -- Pressure Relief Valve/LConn2

== system FuelCellCore/Cathode Gas Channels ==
  Pipe (MA) : fl_lib/Moist Air/Elements/Pipe (MA)  length=sqrt(stack_area) / 2 cm  area=stack_w_channels^2 * stack_num_channels * stack_num_cells cm^2  Dh=stack_w_channels cm  length_add=1 cm  roughness=15e-6 m  Re_lam=2000  Re_tur=4000  shape_factor=64  Nu_lam=3.66  wall_condensation=simscape.enum.onoff.off  RH_ws=1  time_constant=1e-3 s  moisture_trace_gas_source=foundation.enum.moisture_trace_gas_source.none  moisture_source_spec=foundation.enum.moisture_source_spec.vapor  moisture_mass_flow=0 kg/s  moisture_temperature_spec=foundation.enum.temperature_spec.atmospheric  moisture_temperature=293.15 K  trace_gas_mass_flow=0 kg/s  trace_gas_temperature_spec=foundation.enum.temperature_spec.atmospheric  trace_gas_temperature=293.15 K  p_I_specify=on  p_I_priority=High  p_I=env_p MPa  p_I_nominal_specify=off  p_I_nominal_unit=MPa  p_I_nominal_value=1  T_I_specify=on  T_I_priority=High  T_I=env_T degC  T_I_nominal_specify=off  T_I_nominal_unit=K  T_I_nominal_value=1  RH_I_specify=on  RH_I_priority=High  RH_I=env_RH  RH_I_nominal_specify=off  RH_I_nominal_unit=1  RH_I_nominal_value=1  x_w_I_specify=off  x_w_I_priority=None  x_w_I=0  x_w_I_nominal_specify=off  x_w_I_nominal_unit=1  x_w_I_nominal_value=1  y_w_I_specify=off  y_w_I_priority=None  y_w_I=0  y_w_I_nominal_specify=off  y_w_I_nominal_unit=1  y_w_I_nominal_value=1  HR_I_specify=off  HR_I_priority=None  HR_I=0  HR_I_nominal_specify=off  HR_I_nominal_unit=1  HR_I_nominal_value=1  x_g_I_specify=on  x_g_I_priority=None  x_g_I=0  x_g_I_nominal_specify=off  x_g_I_nominal_unit=1  x_g_I_nominal_value=1  y_g_I_specify=on  y_g_I_priority=High  y_g_I=env_yO2  y_g_I_nominal_specify=off  y_g_I_nominal_unit=1  y_g_I_nominal_value=1
  Pipe (MA)1 : fl_lib/Moist Air/Elements/Pipe (MA)  length=sqrt(stack_area) / 2 cm  area=stack_w_channels^2 * stack_num_channels * stack_num_cells cm^2  Dh=stack_w_channels cm  length_add=1 cm  roughness=15e-6 m  Re_lam=2000  Re_tur=4000  shape_factor=64  Nu_lam=3.66  wall_condensation=simscape.enum.onoff.off  RH_ws=1  time_constant=1e-3 s  moisture_trace_gas_source=foundation.enum.moisture_trace_gas_source.controlled  moisture_source_spec=foundation.enum.moisture_source_spec.vapor  moisture_mass_flow=0 kg/s  moisture_temperature_spec=foundation.enum.temperature_spec.atmospheric  moisture_temperature=293.15 K  trace_gas_mass_flow=0 kg/s  trace_gas_temperature_spec=foundation.enum.temperature_spec.atmospheric  trace_gas_temperature=293.15 K  p_I_specify=on  p_I_priority=High  p_I=env_p MPa  p_I_nominal_specify=off  p_I_nominal_unit=MPa  p_I_nominal_value=1  T_I_specify=on  T_I_priority=High  T_I=env_T degC  T_I_nominal_specify=off  T_I_nominal_unit=K  T_I_nominal_value=1  RH_I_specify=on  RH_I_priority=High  RH_I=env_RH  RH_I_nominal_specify=off  RH_I_nominal_unit=1  RH_I_nominal_value=1  x_w_I_specify=off  x_w_I_priority=None  x_w_I=0  x_w_I_nominal_specify=off  x_w_I_nominal_unit=1  x_w_I_nominal_value=1  y_w_I_specify=off  y_w_I_priority=None  y_w_I=0  y_w_I_nominal_specify=off  y_w_I_nominal_unit=1  y_w_I_nominal_value=1  HR_I_specify=off  HR_I_priority=None  HR_I=0  HR_I_nominal_specify=off  HR_I_nominal_unit=1  HR_I_nominal_value=1  x_g_I_specify=on  x_g_I_priority=None  x_g_I=0  x_g_I_nominal_specify=off  x_g_I_nominal_unit=1  x_g_I_nominal_value=1  y_g_I_specify=on  y_g_I_priority=High  y_g_I=env_yO2  y_g_I_nominal_specify=off  y_g_I_nominal_unit=1  y_g_I_nominal_value=1
      settings: InternalSimscapePortConfiguration="{\"Bottom\":[],\"Left\":[{\"id\":\"A\",\"label\":\"A\",\"type\":\"foundation.moist_air.moist_air\"},{\"id\":\"H\",\"label\":\"H\",\"type\":\"foundation.thermal.thermal\"},{\"id\":\"S\",\"label\":\"S\",\"type\":\"foundation.moist_air.moist_air_source\"}],\"Right\":[{\"id\":\"B\",\"label\":\"B\",\"type\":\"foundation.moist_air.moist_air\"},{\"id\":\"W\",\"label\":\"W\",\"type\":\"output\"},{\"id\":\"F\",\"label\":\"F\",\"type\":\"output\"}],\"Top\":[]}"
  C : PMIOPort  Side=Left
  SC : PMIOPort  Port=2  Side=Left
  FCi : PMIOPort  Port=3  Side=Left
  in : PMIOPort  Port=4  Side=Right
  out : PMIOPort  Port=5  Side=Right
  H : PMIOPort  Port=6  Side=Right
  FCo : PMIOPort  Port=7  Side=Left
  connections:
  Pipe (MA)/LConn1 -- in/RConn1
  Pipe (MA)1/RConn1 -- out/RConn1
  Pipe (MA)/LConn2 -- Pipe (MA)1/LConn2 -- H/RConn1
  Pipe (MA)1/RConn3 -- FCo/RConn1
  Pipe (MA)1/LConn3 -- SC/RConn1
  Pipe (MA)/RConn1 -- C/RConn1 -- Pipe (MA)1/LConn1
  Pipe (MA)/RConn3 -- FCi/RConn1
